simulink model "Clutchless_P2_Parallel_ETE"  (R2017b)
settings: Solver=FixedStepAuto  StartTime=0.0  StopTime=length(Speed)  FixedStep=0.01  MaxStep=0.01  RelTol=1e-3  EnableMultiTasking=on
PostLoadFcn:
  | , if any(exist('dsrtsu_mdlpostloadfcn', 'file') == [2, 3, 6]), try dsrtsu_mdlpostloadfcn('Execute', bdroot); catch fprintf('Error in PostLoadFcn (dsrtsu_mdlpostloadfcn) for model "%s":\n %s\n', bdroot, lasterr); end, end,
undefined symbols (not defined in the file): ABSEnable, Actuators, air, APP1_OOR, APP2_OOR, APP_Mismatch, Brk_Flt, cal, ClutchEngag, Clutchless_HSC_ETE, CS_On_Control, Driver, eng, Engine, EngOverTemp, ENGTRQ_MSMCH_Degraded_CP, ENGTRQ_MSMCH_ErrCritical_CP, ENGTRQ_MSMCH_LimpHome_CP, EngTrqMismatch, env, ess, ESSOverTemp, gb, KeyPos_Flt, KeyPosition, lib_Actuators, lib_Clutchless_HSC_ETE, lib_Driver, lib_EMachine_2017a, lib_Sensors_2017a, LossCAN, Machine, max_vehicle_rad_air_flow, MCUOverTemp, mot, MotDirMismatch, MotOverTemp, MotTrqMismatch, mph2ms, PRNDL_Flt, RegenBrkDisable, RegenFault, Sensors, ShiftLeverPosition, Speed, SW_CS_ON, SW_Engine_ON, t_amb, time, tloop
libraries: simulink x97, Pneumatic_lib x11, nesl_utility x9, EC2_libraries x7, powerlib_meascontrol x2, CalculationGallon x1, lib_Chassis x1, lib_DCDC x1, lib_Differential x1, lib_HVESS x1, fl_lib x1, lib_OBC x1
(part 2 of 9)

== system Clutchless_P2_Parallel_ETE/Camaro Plant Model/E-Machine/Soft MCU ==
  In : Inport
  In1 : Inport  Port=2
  Bus Creator : BusCreator  Inputs=5
  Bus Creator1 : BusCreator  Inputs=2
  Bus Selector : BusSelector  OutputSignals=mot_spd_out,mot_trq_out
  Bus Selector1 : BusSelector  OutputSignals=M192_Command_Message.Inverter_Enable,M192_Command_Message.Torque_Command
  Constant : Constant  Value=0
  Data Type Conversion1 : DataTypeConversion
  Data Type Conversion2 : DataTypeConversion
  Data Type Conversion3 : DataTypeConversion
  ForwardDirection : Constant  Value=0
  Memory : Memory
  Subsystem : Subsystem
  Switch : Switch  Criteria=u2 ~= 0  Threshold=1
  Torque Calculation1 : Subsystem
  Torque Calculation2 : Subsystem  Commented=on
  diff_INV_state : MATLAB Function  TreatAsAtomicUnit=on
  diff_INV_state1 : MATLAB Function  TreatAsAtomicUnit=on
  Out : Outport
  Out1 : Outport  Port=2
  wires:
  In1/1 -> Bus Selector/1, Bus Creator1/2  "Sensors_to_MCU"
  Bus Creator1/1 -> Out/1  "MCU_CAN"
  In/1 -> Bus Selector1/1  "HCU_to_MCU"
  Bus Selector1/2 -> Torque Calculation1/1(MotTrqReq)  "<Torque_Command>"
  Bus Creator/1 -> Bus Creator1/1, Out1/1  "MCU_to _Actuator"
  Constant/1 -> Switch/3
  Bus Selector/1 -> Torque Calculation1/2(MotSpd)  "<mot_spd_out>"
  Data Type Conversion1/1 -> Bus Creator/2  "InverterEnabled"
  Bus Selector/2 -> Torque Calculation1/3(MotTrqFdbck), Data Type Conversion2/1  "<mot_trq_out>"
  Data Type Conversion2/1 -> Bus Creator/3  "MotTrqFdbck"
  Memory/1 -> Data Type Conversion1/1
  Switch/1 -> Data Type Conversion3/1  "MotTrqCmd"
  Data Type Conversion3/1 -> Bus Creator/1  "MotTrqCmd"
  ForwardDirection/1 -> Bus Creator/5  "Direction_Command"
  diff_INV_state/1(y) -> diff_INV_state1/1(u)
  Bus Selector1/1 -> Memory/1, diff_INV_state/1(u)  "<Inverter_Enable>"
  diff_INV_state1/1(y) -> Switch/2
  Torque Calculation1/1(mot_trq_out) -> Switch/1
  Subsystem/1(D3_Power_On_Timer) -> Bus Creator/4

== system Clutchless_P2_Parallel_ETE/Camaro Plant Model/ICE Simple1/Engine Plant Modified ==
  "In " : Inport
  eng_spd_out : Inport  Port=2
  Core Engine : Subsystem
      mask Display: image(imread('EngineShortBlock.jpg'),'center')
  ECU Actuators : Subsystem
  ECU Sensors : Subsystem
  Fuel Supply : Subsystem
      mask Display: image(imread('FuelTank.jpg'),'center')
  Radiator : Subsystem
  Subsystem : Subsystem
  Terminator : Terminator
  Terminator1 : Terminator
  eng_shaft_out : Outport
  Out : Outport  Port=2
  tag scope: EngCrankCmd=global, EngRunAtv=global, EngShutdown=global, Eng_Fan=global, Eng_Temp=global, FuelPumpEnable=global, ThrPstCmd_pct=global, VehSpdAvgDrvn_Eng=global
  wires:
  ECU Actuators/5(Out5) -> [EngShutdown]
  Fuel Supply/1(Available Fuel) -> Core Engine/1(Available Fuel)
  ECU Actuators/4(Out4) -> [FuelPumpEnable]
  ECU Actuators/1(Out1) -> [ThrPstCmd_pct]
  "In "/1 -> ECU Actuators/1(In1)
  ECU Actuators/2(Out2) -> [EngCrankCmd]
  ECU Actuators/3(Out3) -> [EngRunAtv]
  Core Engine/1(eng_shaft_out) -> eng_shaft_out/1
  eng_spd_out/1 -> Core Engine/2(Engine Speed (rad/s))
  [Eng_Fan] -> Radiator/2(Fans)
  [Eng_Temp] -> Radiator/1(EngCltTmp)
  ECU Actuators/6(Out6) -> [Eng_Temp]
  ECU Actuators/7(Out7) -> [Eng_Fan]
  ECU Actuators/8(Out8) -> [VehSpdAvgDrvn_Eng]
  Core Engine/2(Throttle Air Flow (g/s)1) -> Terminator/1  "Throttle Air Flow (g/s)"
  [VehSpdAvgDrvn_Eng] -> Terminator1/1
  [EmsCO] -> ECU Sensors/7(In7)  "CO_g/s"
  ECU Sensors/1(Out1) -> Out/1
  [EmsNOx] -> ECU Sensors/9(In9)  "NOx_g/s"
  [FuelLevelPct] -> ECU Sensors/4(In4)  "FuelLevelPct"
  [AdvFuelFlowEst] -> Subsystem/1(EngFuelFlow_g/s), ECU Sensors/3(In3)  "EngFuelFlow_g/s"
  [EmsHC] -> ECU Sensors/6(In6)  "HC_g/s"
  [EngSpd_RPM] -> ECU Sensors/2(In2)  "EngSpd_RPM"
  [EmsCO2] -> ECU Sensors/8(In8)  "CO2_g/s"
  [EngTemp] -> Subsystem/2(Eng_Temp), ECU Sensors/10(In10)  "Eng_Temp"
  [EngPe] -> ECU Sensors/5(In5)  "PE_0_1"
  [EngBrkTrq] -> ECU Sensors/1(In1)  "EngActStdyStTorq_Nm"

== system Clutchless_P2_Parallel_ETE/Camaro Plant Model/ICE Simple1/Inputs ==
  Analog : Subsystem
  Bus Creator : BusCreator  Inputs=2
  CAN_from_HCU : Subsystem
  Inputs : Outport
  wires:
  CAN_from_HCU/1(Out1) -> Bus Creator/1  "CAN"
  Analog/1(Out1) -> Bus Creator/2  "Analog"
  Bus Creator/1 -> Inputs/1

== system Clutchless_P2_Parallel_ETE/Camaro Plant Model/ICE Simple1/Soft ECM ==
  note: Should check lookup table with GM
  In : Inport
  In1 : Inport  Port=2
  Bus Creator1 : BusCreator  Inputs=3
  Bus Creator2 : BusCreator  Inputs=9
  Bus Selector : BusSelector  OutputSignals=EngSpd_RPM
  Bus Selector1 : BusSelector  OutputSignals=Analog.EngAppReq,CAN.to EBCAN.PPEI_Platform_General_Status.SysPwrMd,CAN.to EBCAN.PPEI_Trans_General_Status_2.TrnsShftLvrPos
  Bus Selector2 : BusSelector  OutputSignals=Eng_Temp
  Bus Selector3 : BusSelector  OutputSignals=EngFuelFlow_g/s
  Data Type Conversion : DataTypeConversion  OutDataTypeStr=int8
  Data Type Conversion1 : DataTypeConversion  OutDataTypeStr=int8
  ECM_RollingAliveCnt : Subsystem
  Fuel Consumption : Subsystem
  Logic : Stateflow chart  TreatAsAtomicUnit=on
  Memory1 : Memory  InitialCondition=Engine.Init_T_amb
  Memory2 : Memory
  temp vs fan : Lookup_n-D  NumberOfTableDimensions=1  BreakpointsForDimension1=[0:1:100]  Table=[0:0.01:1]  InternalRulePriority=Speed  RndMeth=Simplest  InputSameDT=on
  Out : Outport
  Out1 : Outport  Port=2
  tag scope: APP_Eng=global, ShiftLvrPos=global
  wires:
  Logic/3(EngRunAtv) -> Bus Creator2/3  "EngRunAtv"
  Bus Selector/1 -> Logic/4(EngSpd_RPM)  "<EngSpd_RPM>"
  Bus Selector1/1 -> Memory2/1  "<EngAppReq>"
  Logic/2(EngCrankCmd) -> Bus Creator2/2  "Eng12vStrtrMtrCmmdOn"
  Bus Creator1/1 -> Out/1  "ECM_CAN"
  Bus Creator2/1 -> Out1/1, Bus Creator1/1  "ECM_to_Actuators"
  Logic/1(ThrottleCmd) -> Bus Creator2/1  "ThrPosCmd_%"
  In1/1 -> Bus Creator1/3, Bus Selector3/1, Bus Selector2/1, Bus Selector/1  "Sensors_to_ECM"
  Logic/4(FuelPumpEnable) -> Bus Creator2/4  "FuelPumpEnable"
  Bus Selector1/2 -> Data Type Conversion/1  "<SysPwrMd>"
  Bus Selector1/3 -> [ShiftLvrPos], Data Type Conversion1/1  "<TrnsShftLvrPos>"
  Logic/5(EngShutdown) -> Bus Creator2/5  "EngShutdown"
  Bus Selector2/1 -> temp vs fan/1, Memory1/1  "<Eng_Temp>"
  Bus Selector3/1 -> Fuel Consumption/1(Fuel Consumption)  "<EngFuelFlow_g/s>"
  Fuel Consumption/1(fuel consumption) -> Bus Creator1/2  "Eng_fuel_consumption"
  temp vs fan/1 -> Bus Creator2/9  "fan_cmd"
  Memory1/1 -> Bus Creator2/8  "Eng_Temp"
  ECM_RollingAliveCnt/1(Out1) -> Bus Creator2/7
  Data Type Conversion/1 -> Logic/2(SysPwrMd)
  Data Type Conversion1/1 -> Logic/3(ShftLvrPos)
  Memory2/1 -> [APP_Eng], Logic/1(drvAPP)
  In/1 -> Bus Selector1/1  "HCU_to_ECM"
  [VehSpdAvgDrvn] -> Bus Creator2/6, Logic/5(VehSpdAvgDrvn)  "VehSpdAvgDrvn"

== system Clutchless_P2_Parallel_ETE/Camaro Plant Model/Scopes/AxlTrq_to_EngTrq2 ==
  note: //From engine axle torque to engine torque//
  In1 : Inport
  Compare To Constant : simulink/Logic and Bit Operations/Compare To Constant  relop===  const=0  OutDataTypeStr=boolean
  Constant1 : Constant  Value=max(gb.plant.init.ratio.map)
  Constant5 : Constant  Value=fd.plant.init.ratio
  Divide1 : Product  Inputs=*//
  Rate Limiter : RateLimiter  RisingSlewLimit=Engine.trq_uprate  FallingSlewLimit=Engine.trq_derate
  Ratio Filter : Subsystem
  Switch : Switch  Criteria=u2 > Threshold
  Out1 : Outport
  wires:
  In1/1 -> Divide1/1
  Constant5/1 -> Divide1/2
  Divide1/1 -> Rate Limiter/1
  [TransRatio] -> Ratio Filter/1(Ratio)
  Compare To Constant/1 -> Switch/2
  Constant1/1 -> Switch/1
  Switch/1 -> Divide1/3
  Rate Limiter/1 -> Out1/1
  Ratio Filter/1(Filtered_Ratio) -> Switch/3, Compare To Constant/1

== system Clutchless_P2_Parallel_ETE/Camaro Plant Model/Scopes/AxlTrq_to_MtrTrq2 ==
  note: //From motor axle torque to motor torque//
  In1 : Inport
  Compare To Constant : simulink/Logic and Bit Operations/Compare To Constant  relop===  const=0  OutDataTypeStr=boolean
  Constant1 : Constant  Value=max(gb.plant.init.ratio.map)
  Constant5 : Constant  Value=fd.plant.init.ratio
  Divide : Product  Inputs=*//
  Rate Limiter : RateLimiter  RisingSlewLimit=mcu.plant.init.trq_uprate  FallingSlewLimit=mcu.plant.init.trq_derate
  Ratio Filter : Subsystem
  Switch : Switch  Criteria=u2 > Threshold
  Out1 : Outport
  wires:
  In1/1 -> Divide/1
  Constant5/1 -> Divide/2
  Divide/1 -> Rate Limiter/1
  [TransRatio] -> Ratio Filter/1(Ratio)
  Compare To Constant/1 -> Switch/2
  Constant1/1 -> Switch/1
  Rate Limiter/1 -> Out1/1
  Switch/1 -> Divide/3
  Ratio Filter/1(Filtered_Ratio) -> Switch/3, Compare To Constant/1

== system Clutchless_P2_Parallel_ETE/Clutchless_HSC_ETE/HSC/Camaro Fault Detection ==
  Sensors : Inport
  Component Diagnostic : Subsystem
  Input Conversions : Subsystem
  Signal Diagnostic : Subsystem
  SystemDiag : lib_SystemDiag/SystemDiag
  Diagnostic : Outport
  wires:
  Signal Diagnostic/1(SignalDiag) -> Component Diagnostic/1(SignalDiag)
  Component Diagnostic/1(CompDiag) -> SystemDiag/1
  Input Conversions/1(VehSig) -> Signal Diagnostic/1(VehSig)
  Sensors/1 -> Input Conversions/1(RawSig)
  SystemDiag/1 -> Diagnostic/1

== system Clutchless_P2_Parallel_ETE/Clutchless_HSC_ETE/HSC/Driver_Requests ==
  note: Driver management
  Sensors : Inport
  "Diagnostic " : Inport  Port=2
  "Controls " : Inport  Port=3
  APP_BPP to DrvIntndAxlTrq2 : Subsystem
  DriverRequests : Outport
  wires:
  "Controls "/1 -> APP_BPP to DrvIntndAxlTrq2/3(Controls)
  "Diagnostic "/1 -> APP_BPP to DrvIntndAxlTrq2/2(Diag)
  APP_BPP to DrvIntndAxlTrq2/1(IntndAxlTrq) -> DriverRequests/1
  Sensors/1 -> APP_BPP to DrvIntndAxlTrq2/1(Sensors)

== system Clutchless_P2_Parallel_ETE/Clutchless_HSC_ETE/HSC/Powertrain Manager ==
  Sensors : Inport
  Driver Request : Inport  Port=2
  Fault Detection : Inport  Port=3
  Ground : Ground
  HV Manager1 : Subsystem  AncestorBlock=lib_HVManager_PostIMG_2017a/HV Manager
  Output Conversion : Subsystem
  Thermal Manager : Subsystem  AncestorBlock=lib_ThermalManager/Thermal Manager
  Torque Distribution : Subsystem  AncestorBlock=lib_TorqueDistribution_2017a/Torque Distribution
  Out1 : Outport
  Controls : Outport  Port=2
  tag scope: HV_BUS_Status=global
  wires:
  Torque Distribution/1(Controls) -> [Controls], Controls/1, HV Manager1/2(Controls)
  Ground/1 -> Output Conversion/9(In11)  "Trans_test"
  HV Manager1/1(BMS_CAN) -> [BMS_CAN]
  HV Manager1/2(HV_BUS_Status) -> [HV_BUS_Status]
  HV Manager1/4(OBC_Digital) -> [OBC_Digital]
  HV Manager1/3(OBC_CAN) -> [OBC_CAN]
  Driver Request/1 -> Torque Distribution/2(Driver Request)
  [BMS_CAN] -> Output Conversion/1(In1)  "BMS_CAN"
  [OBC_CAN] -> Output Conversion/2(In2)  "OBC_CAN"
  [MCU_CAN] -> Output Conversion/3(In3)  "MCU_CAN"
  [Controls] -> Output Conversion/4(In4)  "Controls"
  Output Conversion/1(Out1) -> Out1/1
  HV Manager1/5(BMS_Digital) -> [BMS_Digital]
  [BMS_Digital] -> Output Conversion/5(In5)  "BMS_Digital"
  Fault Detection/1 -> Torque Distribution/3(Fault Detection)
  Thermal Manager/1(Out1) -> [Fuel_Pump_Control]
  HV Manager1/6(Axiomatic_CAN) -> [Axiomatic_CAN]
  [Axiomatic_CAN] -> Output Conversion/8(In10)  "Axiomatic_CAN"
  [OBC_Digital] -> Output Conversion/7(In9)  "OBC_Digital"
  [Fuel_Pump_Control] -> Output Conversion/6(In8)  "Fuel_Pump_Control"
  Sensors/1 -> Thermal Manager/1(In2), HV Manager1/1(Sensors), Torque Distribution/1(Sensors)

== system Clutchless_P2_Parallel_ETE/Driver/Driver Control/Override CS SW ==
  note: This subsystem is used to override the model value of a signal to a constant value
  note: Override Switch Subsystem
  In1 : Inport
  Multiport Switch : MultiPortSwitch  DataPortOrder=Zero-based contiguous  Inputs=2  zeroidx=on
  Override Value : Constant  Value=0  OutDataTypeStr=double
  Signal Override Switch 0 = Use Model 1 = Use Constant : Constant
  Out1 : Outport
  wires:
  Signal Override Switch 0 = Use Model 1 = Use Constant/1 -> Multiport Switch/1
  In1/1 -> Multiport Switch/2
  Multiport Switch/1 -> Out1/1
  Override Value/1 -> Multiport Switch/3

== system Clutchless_P2_Parallel_ETE/Driver/Driver Control/Override Engine SW ==
  note: Override Switch Subsystem
  note: This subsystem is used to override the model value of a signal to a constant value
  In1 : Inport
  Multiport Switch : MultiPortSwitch  DataPortOrder=Zero-based contiguous  Inputs=2  zeroidx=on
  Override Value : Constant  Value=0  OutDataTypeStr=double
  Signal Override Switch 0 = Use Model 1 = Use Constant : Constant
  Out1 : Outport
  wires:
  Override Value/1 -> Multiport Switch/3
  Multiport Switch/1 -> Out1/1
  In1/1 -> Multiport Switch/2
  Signal Override Switch 0 = Use Model 1 = Use Constant/1 -> Multiport Switch/1

== system Clutchless_P2_Parallel_ETE/Driver/Driver Control/Override Regen SW ==
  note: This subsystem is used to override the model value of a signal to a constant value
  note: Override Switch Subsystem
  In1 : Inport
  Multiport Switch : MultiPortSwitch  DataPortOrder=Zero-based contiguous  Inputs=2  zeroidx=on
  Override Value : Constant  Value=0  OutDataTypeStr=double
  Signal Override Switch 0 = Use Model 1 = Use Constant : Constant
  Out1 : Outport
  wires:
  Signal Override Switch 0 = Use Model 1 = Use Constant/1 -> Multiport Switch/1
  In1/1 -> Multiport Switch/2
  Multiport Switch/1 -> Out1/1
  Override Value/1 -> Multiport Switch/3

== system Clutchless_P2_Parallel_ETE/Fault Trigger /Component Diagnostics setting/Mismch type ==
  In1 : Inport
  Constant : Constant  Value=cal.ENGTRQ_MSMCH.Degraded_CP+1
  Constant1 : Constant  Value=cal.ENGTRQ_MSMCH.LimpHome_CP+1
  Constant2 : Constant  Value=cal.ENGTRQ_MSMCH.ErrCritical_CP+1
  Constant3 : Constant  Value=0
  Multiport Switch : MultiPortSwitch  DataPortOrder=Zero-based contiguous  Inputs=4
  Out1 : Outport
  wires:
  Constant1/1 -> Multiport Switch/4
  Constant2/1 -> Multiport Switch/5
  In1/1 -> Multiport Switch/1
  Multiport Switch/1 -> Out1/1
  Constant3/1 -> Multiport Switch/2
  Constant/1 -> Multiport Switch/3

== system Clutchless_P2_Parallel_ETE/Fault Trigger /Component Diagnostics setting/Mismch type1 ==
  In1 : Inport
  Constant : Constant  Value=cal.MOTTRQ_MSMCH.Degraded_CP+1
  Constant1 : Constant  Value=cal.MOTTRQ_MSMCH.LimpHome_CP+1
  Constant2 : Constant  Value=cal.ENGTRQ_MSMCH.ErrCritical_CP+1
  Constant3 : Constant  Value=0
  Multiport Switch : MultiPortSwitch  DataPortOrder=Zero-based contiguous  Inputs=4
  Out1 : Outport
  wires:
  Constant/1 -> Multiport Switch/3
  Constant3/1 -> Multiport Switch/2
  Multiport Switch/1 -> Out1/1
  In1/1 -> Multiport Switch/1
  Constant2/1 -> Multiport Switch/5
  Constant1/1 -> Multiport Switch/4

== system Clutchless_P2_Parallel_ETE/Fault Trigger /Component Diagnostics setting/Override  ClutchEngag ==
  note: Override Switch Subsystem
  note: This subsystem is used to override the model value of a signal to a constant value
  In1 : Inport
  Constant : Constant  Value=0
  Multiport Switch : MultiPortSwitch  DataPortOrder=Zero-based contiguous  Inputs=2
  Signal Override Switch 0 = Use Model 1 = Use Constant : Constant  Value=ClutchEngagFlt
  Out1 : Outport
  wires:
  Constant/1 -> Multiport Switch/3
  Multiport Switch/1 -> Out1/1
  In1/1 -> Multiport Switch/2
  Signal Override Switch 0 = Use Model 1 = Use Constant/1 -> Multiport Switch/1

== system Clutchless_P2_Parallel_ETE/Fault Trigger /Component Diagnostics setting/Override  ESSOverTemp ==
  note: This subsystem is used to override the model value of a signal to a constant value
  note: Override Switch Subsystem
  In1 : Inport
  Constant : Constant  Value=0
  Multiport Switch : MultiPortSwitch  DataPortOrder=Zero-based contiguous  Inputs=2
  Signal Override Switch 0 = Use Model 1 = Use Constant : Constant  Value=ESSOverTemp_ON
  Out1 : Outport
  wires:
  Signal Override Switch 0 = Use Model 1 = Use Constant/1 -> Multiport Switch/1
  In1/1 -> Multiport Switch/2
  Multiport Switch/1 -> Out1/1
  Constant/1 -> Multiport Switch/3

== system Clutchless_P2_Parallel_ETE/Fault Trigger /Component Diagnostics setting/Override  EngOverTemp ==
  note: Override Switch Subsystem
  note: This subsystem is used to override the model value of a signal to a constant value
  In1 : Inport
  Constant : Constant  Value=0
  Multiport Switch : MultiPortSwitch  DataPortOrder=Zero-based contiguous  Inputs=2
  Signal Override Switch 0 = Use Model 1 = Use Constant : Constant  Value=EngOverTemp_ON
  Out1 : Outport
  wires:
  Constant/1 -> Multiport Switch/3
  Multiport Switch/1 -> Out1/1
  In1/1 -> Multiport Switch/2
  Signal Override Switch 0 = Use Model 1 = Use Constant/1 -> Multiport Switch/1

== system Clutchless_P2_Parallel_ETE/Fault Trigger /Component Diagnostics setting/Override  EngTrqMismatch ==
  note: This subsystem is used to override the model value of a signal to a constant value
  note: Override Switch Subsystem
  In1 : Inport
  Constant : Constant  Value=0
  Multiport Switch : MultiPortSwitch  DataPortOrder=Zero-based contiguous  Inputs=2
  Signal Override Switch 0 = Use Model 1 = Use Constant : Constant  Value=EngTrqMismatch_ON
  Out1 : Outport
  wires:
  Signal Override Switch 0 = Use Model 1 = Use Constant/1 -> Multiport Switch/1
  In1/1 -> Multiport Switch/2
  Multiport Switch/1 -> Out1/1
  Constant/1 -> Multiport Switch/3

== system Clutchless_P2_Parallel_ETE/Fault Trigger /Component Diagnostics setting/Override  LossCAN ==
  note: Override Switch Subsystem
  note: This subsystem is used to override the model value of a signal to a constant value
  In1 : Inport
  Constant : Constant  Value=0
  Multiport Switch : MultiPortSwitch  DataPortOrder=Zero-based contiguous  Inputs=2
  Signal Override Switch 0 = Use Model 1 = Use Constant : Constant  Value=LossCAN_ON
  Out1 : Outport
  wires:
  Constant/1 -> Multiport Switch/3
  Multiport Switch/1 -> Out1/1
  In1/1 -> Multiport Switch/2
  Signal Override Switch 0 = Use Model 1 = Use Constant/1 -> Multiport Switch/1

== system Clutchless_P2_Parallel_ETE/Fault Trigger /Component Diagnostics setting/Override  MCUOverTemp ==
  note: This subsystem is used to override the model value of a signal to a constant value
  note: Override Switch Subsystem
  In1 : Inport
  Constant : Constant  Value=0
  Multiport Switch : MultiPortSwitch  DataPortOrder=Zero-based contiguous  Inputs=2
  Signal Override Switch 0 = Use Model 1 = Use Constant : Constant  Value=MCUOverTemp_ON
  Out1 : Outport
  wires:
  Signal Override Switch 0 = Use Model 1 = Use Constant/1 -> Multiport Switch/1
  In1/1 -> Multiport Switch/2
  Multiport Switch/1 -> Out1/1
  Constant/1 -> Multiport Switch/3

== system Clutchless_P2_Parallel_ETE/Fault Trigger /Component Diagnostics setting/Override  MotDirMismatch ==
  note: Override Switch Subsystem
  note: This subsystem is used to override the model value of a signal to a constant value
  In1 : Inport
  Constant : Constant  Value=0
  Multiport Switch : MultiPortSwitch  DataPortOrder=Zero-based contiguous  Inputs=2
  Signal Override Switch 0 = Use Model 1 = Use Constant : Constant  Value=MotDirMismatch_ON
  Out1 : Outport
  wires:
  Constant/1 -> Multiport Switch/3
  Multiport Switch/1 -> Out1/1
  In1/1 -> Multiport Switch/2
  Signal Override Switch 0 = Use Model 1 = Use Constant/1 -> Multiport Switch/1

== system Clutchless_P2_Parallel_ETE/Fault Trigger /Component Diagnostics setting/Override  MotOverTemp ==
  note: Override Switch Subsystem
  note: This subsystem is used to override the model value of a signal to a constant value
  In1 : Inport
  Constant : Constant  Value=0
  Multiport Switch : MultiPortSwitch  DataPortOrder=Zero-based contiguous  Inputs=2
  Signal Override Switch 0 = Use Model 1 = Use Constant : Constant  Value=MotOverTemp_ON
  Out1 : Outport
  wires:
  Constant/1 -> Multiport Switch/3
  Multiport Switch/1 -> Out1/1
  In1/1 -> Multiport Switch/2
  Signal Override Switch 0 = Use Model 1 = Use Constant/1 -> Multiport Switch/1

== system Clutchless_P2_Parallel_ETE/Fault Trigger /Component Diagnostics setting/Override  MotTrqMismatch ==
  note: This subsystem is used to override the model value of a signal to a constant value
  note: Override Switch Subsystem
  In1 : Inport
  Constant : Constant  Value=0
  Multiport Switch : MultiPortSwitch  DataPortOrder=Zero-based contiguous  Inputs=2
  Signal Override Switch 0 = Use Model 1 = Use Constant : Constant  Value=MotTrqMismatch_ON
  Out1 : Outport
  wires:
  Signal Override Switch 0 = Use Model 1 = Use Constant/1 -> Multiport Switch/1
  In1/1 -> Multiport Switch/2
  Multiport Switch/1 -> Out1/1
  Constant/1 -> Multiport Switch/3

== system Clutchless_P2_Parallel_ETE/Fault Trigger /Driver Interface Diagnostics setting/Override  APP1_OOR ==
  note: Signal Override Switch
      | 0 = Use Model
      | 1 = Use Constant
  note: Override Switch Subsystem
  note: This subsystem is used to override the model value of a signal to a constant value
  In1 : Inport
  APP1_OOR_ON : Constant  Value=APP1_OOR_ON
  Constant : Constant  Value=0
  Multiport Switch : MultiPortSwitch  DataPortOrder=Zero-based contiguous  Inputs=2
  Out1 : Outport
  wires:
  Constant/1 -> Multiport Switch/3
  Multiport Switch/1 -> Out1/1
  In1/1 -> Multiport Switch/2
  APP1_OOR_ON/1 -> Multiport Switch/1

== system Clutchless_P2_Parallel_ETE/Fault Trigger /Driver Interface Diagnostics setting/Override  APP2_OOR ==
  note: Signal Override Switch
      | 0 = Use Model
      | 1 = Use Constant
  note: This subsystem is used to override the model value of a signal to a constant value
  note: Override Switch Subsystem
  In1 : Inport
  APP2_OOR_ON : Constant  Value=APP2_OOR_ON
  Constant : Constant  Value=0
  Multiport Switch : MultiPortSwitch  DataPortOrder=Zero-based contiguous  Inputs=2
  Out1 : Outport
  wires:
  APP2_OOR_ON/1 -> Multiport Switch/1
  In1/1 -> Multiport Switch/2
  Multiport Switch/1 -> Out1/1
  Constant/1 -> Multiport Switch/3

== system Clutchless_P2_Parallel_ETE/Fault Trigger /Driver Interface Diagnostics setting/Override  APP_Mismatch ==
  note: Signal Override Switch
      | 0 = Use Model
      | 1 = Use Constant
  note: Override Switch Subsystem
  note: This subsystem is used to override the model value of a signal to a constant value
  In1 : Inport
  APP_Mismatch_Override : Constant  Value=Mismatch_APP_ON
  Constant : Constant  Value=0
  Multiport Switch : MultiPortSwitch  DataPortOrder=Zero-based contiguous  Inputs=2
  Out1 : Outport
  wires:
  Constant/1 -> Multiport Switch/3
  Multiport Switch/1 -> Out1/1
  In1/1 -> Multiport Switch/2
  APP_Mismatch_Override/1 -> Multiport Switch/1

== system Clutchless_P2_Parallel_ETE/Fault Trigger /Driver Interface Diagnostics setting/Override  BPP_Flt ==
  note: Signal Override Switch
      | 0 = Use Model
      | 1 = Use Constant
  note: This subsystem is used to override the model value of a signal to a constant value
  note: Override Switch Subsystem
  In1 : Inport
  Brk_Flt_ON : Constant  Value=Brk_Flt_ON
  Constant : Constant  Value=0
  Multiport Switch : MultiPortSwitch  DataPortOrder=Zero-based contiguous  Inputs=2
  Out1 : Outport
  wires:
  Brk_Flt_ON/1 -> Multiport Switch/1
  In1/1 -> Multiport Switch/2
  Multiport Switch/1 -> Out1/1
  Constant/1 -> Multiport Switch/3

== system Clutchless_P2_Parallel_ETE/Fault Trigger /Driver Interface Diagnostics setting/Override  KeyPos_Flt ==
  note: Signal Override Switch
      | 0 = Use Model
      | 1 = Use Constant
  note: Override Switch Subsystem
  note: This subsystem is used to override the model value of a signal to a constant value
  In1 : Inport
  Constant : Constant  Value=0
  KeyPos_Flt_ON : Constant  Value=KeyPos_Flt_ON
  Multiport Switch : MultiPortSwitch  DataPortOrder=Zero-based contiguous  Inputs=2
  Out1 : Outport
  wires:
  Constant/1 -> Multiport Switch/3
  Multiport Switch/1 -> Out1/1
  In1/1 -> Multiport Switch/2
  KeyPos_Flt_ON/1 -> Multiport Switch/1

== system Clutchless_P2_Parallel_ETE/Fault Trigger /Driver Interface Diagnostics setting/Override  PRNDL_Flt ==
  note: Signal Override Switch
      | 0 = Use Model
      | 1 = Use Constant
  note: This subsystem is used to override the model value of a signal to a constant value
  note: Override Switch Subsystem
  In1 : Inport
  Constant : Constant  Value=0
  Multiport Switch : MultiPortSwitch  DataPortOrder=Zero-based contiguous  Inputs=2
  PRNDL_Flt_ON : Constant  Value=PRNDL_Flt_ON
  Out1 : Outport
  wires:
  PRNDL_Flt_ON/1 -> Multiport Switch/1
  In1/1 -> Multiport Switch/2
  Multiport Switch/1 -> Out1/1
  Constant/1 -> Multiport Switch/3

== system Clutchless_P2_Parallel_ETE/Sensors/CAN/EBCAN ==
  In1 : Inport
  BMS_Antrieb : Subsystem
  Bus Creator : BusCreator  Inputs=3
  Bus Selector : BusSelector  OutputSignals=ECM_CAN,BMS_CAN.BMS_Hybrid
  CCM : Subsystem
  ECM : Subsystem
  Out1 : Outport
  wires:
  Bus Selector/2 -> CCM/1(In1), BMS_Antrieb/1(In1)  "<BMS_Hybrid>"
  Bus Selector/1 -> ECM/1(In1)  "<ECM_CAN>"
  In1/1 -> Bus Selector/1
  CCM/1(Out1) -> Bus Creator/3  "from_CCM"
  Bus Creator/1 -> Out1/1
  BMS_Antrieb/1(Out1) -> Bus Creator/2  "from_BMSAntrieb"
  ECM/1(Out1) -> Bus Creator/1  "from_ECM"

== system Clutchless_P2_Parallel_ETE/Sensors/CAN/HV_CAN ==
  In1 : Inport
  BMS_Hybrid : Subsystem
  Bus Creator : BusCreator  Inputs=3
  Bus Selector : BusSelector  OutputSignals=MCU_CAN,BMS_CAN.BMS_Plugin,OBC_CAN
  MCU : Subsystem
  OBC : Subsystem
  Out1 : Outport
  wires:
  Bus Selector/3 -> OBC/1(In1)  "<OBC_CAN>"
  Bus Selector/2 -> BMS_Hybrid/1(In1)  "<BMS_Plugin>"
  Bus Selector/1 -> MCU/1(In1)  "<MCU_CAN>"
  In1/1 -> Bus Selector/1
  Bus Creator/1 -> Out1/1
  OBC/1(Out1) -> Bus Creator/3  "from_OBC"
  BMS_Hybrid/1(Out1) -> Bus Creator/2  "from_BMSHybrid"
  MCU/1(Out1) -> Bus Creator/1  "from_MCU"

== system Clutchless_P2_Parallel_ETE/Sensors/CAN/VEH_CAN ==
  In1 : Inport
  BCM : Subsystem
  Bus Creator : BusCreator  Inputs=4
  Bus Selector : BusSelector  OutputSignals=TCM_CAN,BCM_CAN
  EBCM : Subsystem  Commented=on
  Ground : Ground  Commented=on
  Ground1 : Ground  Commented=on
  ICCM : Subsystem  Commented=on
  TCM : Subsystem
  Out1 : Outport
  wires:
  Ground/1 -> EBCM/1(In1)  "<EBCM>"
  Ground1/1 -> ICCM/1(In1)  "<ONSTAR>"
  Bus Selector/2 -> BCM/1(In1)  "<BCM_CAN>"
  Bus Selector/1 -> TCM/1(In1)  "<TCM_CAN>"
  Bus Creator/1 -> Out1/1
  EBCM/1(Out1) -> Bus Creator/4  "from_EBCM"
  ICCM/1(Out1) -> Bus Creator/3  "from_ICCM"
  BCM/1(Out1) -> Bus Creator/2  "from_BCM"
  TCM/1(Out1) -> Bus Creator/1  "from_TCM"
  In1/1 -> Bus Selector/1

== system Clutchless_P2_Parallel_ETE/Actuators/CAN/EBCAN/ISO_Hybrid_01_Req ==
  In1 : Inport
  Bus Creator : BusCreator  Inputs=1
  Bus Selector : BusSelector  OutputSignals=ISO_Hybrid_01_Req_Data_byte_3
  Data Type Conversion : DataTypeConversion
  Out1 : Outport
  wires:
  In1/1 -> Bus Selector/1
  Data Type Conversion/1 -> Bus Creator/1  "ISO_Hybrid_01_Req_Data_4"
  Bus Creator/1 -> Out1/1  "ISO_Hybrid_01_Req"
  Bus Selector/1 -> Data Type Conversion/1  "<ISO_Hybrid_01_Req_Data_byte_3>"

== system Clutchless_P2_Parallel_ETE/Actuators/CAN/EBCAN/PPEI_Platform_General_Status ==
  In1 : Inport
  Bus Creator : BusCreator  Inputs=1
  Data Type Conversion : DataTypeConversion
  Out1 : Outport
  wires:
  Bus Creator/1 -> Out1/1  "PPEI_Platform_General_Status"
  Data Type Conversion/1 -> Bus Creator/1  "SysPwrMd"
  In1/1 -> Data Type Conversion/1

== system Clutchless_P2_Parallel_ETE/Actuators/CAN/EBCAN/PPEI_Trans_General_Status_2 ==
  In1 : Inport
  Bus Creator : BusCreator  Inputs=1
  Data Type Conversion : DataTypeConversion
  Out1 : Outport
  wires:
  In1/1 -> Data Type Conversion/1
  Data Type Conversion/1 -> Bus Creator/1  "TrnsShftLvrPos"
  Bus Creator/1 -> Out1/1  "PPEI_Trans_General_Status_2"

== system Clutchless_P2_Parallel_ETE/Actuators/CAN/VEH_CAN/BCM ==
  In1 : Inport
  Bus Creator : BusCreator  Inputs=1
  Bus Selector : BusSelector  OutputSignals=Controls.powerMode
  Out1 : Outport
  wires:
  In1/1 -> Bus Selector/1
  Bus Selector/1 -> Bus Creator/1  "<powerMode>"
  Bus Creator/1 -> Out1/1

== system Clutchless_P2_Parallel_ETE/Actuators/CAN/VEH_CAN/EBCM ==
  In1 : Inport
  Out1 : Outport
  wires:
  In1/1 -> Out1/1

== system Clutchless_P2_Parallel_ETE/Actuators/CAN/VEH_CAN/ICCM ==
  In1 : Inport
  Out1 : Outport
  wires:
  In1/1 -> Out1/1

== system Clutchless_P2_Parallel_ETE/Camaro Plant Model/E-Machine/IMG Plant/ Actuators ==
  In1 : Inport
  Bus Selector : BusSelector  OutputSignals=MotTrqCmd,Direction_Command,InverterEnabled
  MotTrqCmd : Outport
  DirectionCommand : Outport  Port=2
  InverterEnabled : Outport  Port=3
  wires:
  In1/1 -> Bus Selector/1
  Bus Selector/1 -> MotTrqCmd/1  "<MotTrqCmd>"
  Bus Selector/2 -> DirectionCommand/1  "<Direction_Command>"
  Bus Selector/3 -> InverterEnabled/1  "<InverterEnabled>"

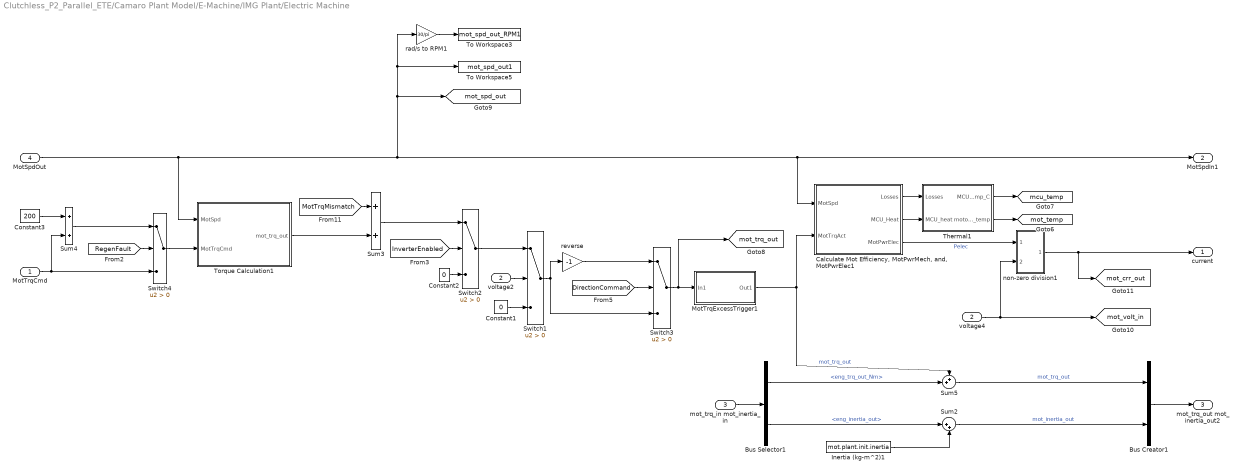
== system Clutchless_P2_Parallel_ETE/Camaro Plant Model/E-Machine/IMG Plant/Electric Machine ==
  MotTrqCmd : Inport
  voltage2 : Inport  Port=2
  mot_trq_in mot_inertia_in : Inport  Port=3
  MotSpdOut : Inport  Port=4
  Bus Creator1 : BusCreator  Inputs=2
  Bus Selector1 : BusSelector  OutputSignals=eng_trq_out_Nm,eng_inertia_out
  "Calculate Mot Efficiency, MotPwrMech, and, MotPwrElec1" : Subsystem
  Constant1 : Constant  Value=0
  Constant2 : Constant  Value=0
  Constant3 : Constant  Value=200
  Inertia (kg-m^2)1 : Constant  Value=mot.plant.init.inertia
  MotTrqExcessTrigger1 : Subsystem
  Sum2 : Sum  Inputs=|++
  Sum3 : Sum
  Sum4 : Sum
  Sum5 : Sum  Inputs=++|
  Switch{1..4} (4 alike) : Switch  Criteria=u2 > Threshold
  Thermal1 : Subsystem
  To Workspace3 : ToWorkspace  VariableName=mot_spd_out_RPM1  SampleTime=-1
      settings: Decimation=WORKSPACE_DECIMATION
  To Workspace5 : ToWorkspace  VariableName=mot_spd_out1  SampleTime=-1
      settings: Decimation=WORKSPACE_DECIMATION
  Torque Calculation1 : Subsystem
  non-zero division1 : Subsystem
      mask Display: disp('divider \n I1/I2')
  rad/s to RPM1 : Gain  Gain=30/pi
  reverse : Gain  Gain=-1
  voltage4 : InportShadow  Port=2
  current : Outport
  MotSpdIn1 : Outport  Port=2
  mot_trq_out mot_inertia_out2 : Outport  Port=3
  tag scope: mcu_temp=global, mot_crr_out=global, mot_spd_out=global, mot_temp=global, mot_trq_out=global, mot_volt_in=global
  wires:
  Thermal1/1(MCU_temp_C) -> [mcu_temp]
  Thermal1/2(motor_temp) -> [mot_temp]
  Constant3/1 -> Sum4/1
  Torque Calculation1/1(mot_trq_out) -> Sum3/2
  Switch2/1 -> Switch1/1
  [RegenFault] -> Switch4/2
  "Calculate Mot Efficiency, MotPwrMech, and, MotPwrElec1"/1(Losses) -> Thermal1/1(Losses)
  Sum4/1 -> Switch4/1
  Switch3/1 -> MotTrqExcessTrigger1/1(In1), [mot_trq_out]
  "Calculate Mot Efficiency, MotPwrMech, and, MotPwrElec1"/2(MCU_Heat) -> Thermal1/2(MCU_heat)
  Switch4/1 -> Torque Calculation1/2(MotTrqCmd)
  "Calculate Mot Efficiency, MotPwrMech, and, MotPwrElec1"/3(MotPwrElec) -> non-zero division1/1(In1)  "Pelec"
  reverse/1 -> Switch3/1
  non-zero division1/1(Out1) -> [mot_crr_out], current/1
  MotTrqExcessTrigger1/1(Out1) -> Sum5/1, "Calculate Mot Efficiency, MotPwrMech, and, MotPwrElec1"/2(MotTrqAct)  "mot_trq_out"
  Sum3/1 -> Switch2/1
  MotTrqCmd/1 -> Sum4/2, Switch4/3
  Constant2/1 -> Switch2/3
  Switch1/1 -> reverse/1, Switch3/3
  Constant1/1 -> Switch1/3
  voltage2/1 -> Switch1/2
  voltage4/1 -> non-zero division1/2(In2), [mot_volt_in]
  [MotTrqMismatch] -> Sum3/1
  [InverterEnabled] -> Switch2/2
  [DirectionCommand] -> Switch3/2
  Sum5/1 -> Bus Creator1/1  "mot_trq_out"
  Inertia (kg-m^2)1/1 -> Sum2/2
  Sum2/1 -> Bus Creator1/2  "mot_inertia_out"
  Bus Creator1/1 -> mot_trq_out mot_inertia_out2/1
  mot_trq_in mot_inertia_in/1 -> Bus Selector1/1
  Bus Selector1/2 -> Sum2/1  "<eng_inertia_out>"
  Bus Selector1/1 -> Sum5/2  "<eng_trq_out_Nm>"
  rad/s to RPM1/1 -> To Workspace3/1
  MotSpdOut/1 -> "Calculate Mot Efficiency, MotPwrMech, and, MotPwrElec1"/1(MotSpd), MotSpdIn1/1, To Workspace5/1, rad/s to RPM1/1, [mot_spd_out], Torque Calculation1/1(MotSpd)

== system Clutchless_P2_Parallel_ETE/Camaro Plant Model/E-Machine/IMG Plant/Sensors ==
  In2 : Inport
  In3 : Inport  Port=2
  In4 : Inport  Port=3
  In5 : Inport  Port=4
  In6 : Inport  Port=5
  In1 : Inport  Port=6
  In7 : Inport  Port=7
  Bus Creator : BusCreator  Inputs=7
  Out1 : Outport
  wires:
  Bus Creator/1 -> Out1/1
  In2/1 -> Bus Creator/1  "mot_spd_out"
  In4/1 -> Bus Creator/3  "mot_crr_out"
  In5/1 -> Bus Creator/4  "mot_volt_in"
  In3/1 -> Bus Creator/2  "mot_trq_out"
  In6/1 -> Bus Creator/5  "mot_temp"
  In1/1 -> Bus Creator/6  "mcu_temp"
  In7/1 -> Bus Creator/7  "clt_plant_spd_in"

== system Clutchless_P2_Parallel_ETE/Camaro Plant Model/E-Machine/IMG Plant2/ Actuators ==
  In1 : Inport
  Bus Selector : BusSelector  OutputSignals=MotTrqCmd,Direction_Command,InverterEnabled
  Out2 : Outport
  Out3 : Outport  Port=2
  Out4 : Outport  Port=3
  wires:
  Bus Selector/3 -> Out4/1  "<InverterEnabled>"
  Bus Selector/2 -> Out3/1  "<Direction_Command>"
  In1/1 -> Bus Selector/1
  Bus Selector/1 -> Out2/1  "<MotTrqCmd>"

== system Clutchless_P2_Parallel_ETE/Camaro Plant Model/E-Machine/IMG Plant2/Calculate Mot Efficiency, MotPwrMech, and, MotPwrElec ==
  note: Pelec_req = Pmech_req*Eff^k,
      | k = -1 if Trq >= 0,
      | k = 1 if Trq < 0
  MotSpd : Inport
  MotTrqAct : Inport  Port=2
  -1 : Gain  Gain=8
  "-1 when + 1 when - " : Gain  Gain=-1
  -2 : Gain  Gain=tloop
  2-D Lookup Table : Lookup_n-D  BreakpointsForDimension1=mot.plant.init.eff_trq.idx2_trq  BreakpointsForDimension2=mot.plant.init.eff_trq.idx1_spd  Table=mot.plant.init.eff_trq.map  InternalRulePriority=Speed  RndMeth=Simplest  InputSameDT=on
  Abs{,1..3} (4 alike) : Abs
  Add : Sum  Inputs=-+
  Add1 : Sum  Inputs=+-
  Add2 : Sum  Commented=on
  Constant : Constant  Value=1-0.8
  Constant1 : Constant  Commented=on  Value=mot.plant.init.mcu_mass
  Constant2 : Constant  Commented=on  Value=mot.plant.init.specific_heat
  Divide : Product  Commented=on  Inputs=*/
  Gain2 : Gain  Gain=1/100
  Lower Limit : Subsystem  Commented=on  mask{Lolimit=t_amb+20}
      mask prompts: Lolimit "Lower Limit"
  MCUOverTemp Fault : Subsystem  Commented=on
  MCU_WEGPmp : Constant  Value=0
  Math Function1 : Math  Operator=pow  SaturateOnIntegerOverflow=on
  Memory : Memory
  Memory1 : Memory  Commented=on
  Product : Product
  Product1 : Product
  Product2 : Product
  Product3 : Product  Commented=on
  Sign : Signum
  rad/s to rpm : Gain  Gain=30/pi
  Losses : Outport
  MotPwrElec : Outport  Port=2
  MCU_Heat : Outport  Port=3
  wires:
  Lower Limit/1(Out1) -> Memory1/1, MCUOverTemp Fault/1(In1)
  Add2/1 -> Lower Limit/1(In1)
  Memory1/1 -> Add2/2
  Divide/1 -> Add2/1
  Product3/1 -> Divide/2
  Constant2/1 -> Product3/2
  Constant1/1 -> Product3/1
  -2/1 -> MCU_Heat/1
  -1/1 -> Add1/2
  Add1/1 -> -2/1
  MCU_WEGPmp/1 -> -1/1
  Abs3/1 -> Add1/1
  Product2/1 -> Abs3/1
  Constant/1 -> Product2/2
  Memory/1 -> Sign/1
  Math Function1/1 -> Product1/2
  Add/1 -> Abs2/1
  Abs2/1 -> Losses/1
  "-1 when + 1 when - "/1 -> Math Function1/2
  MotSpd/1 -> rad/s to rpm/1, Product/2
  MotTrqAct/1 -> Abs/1, Product/1, Memory/1
  Product/1 -> Product1/1, Add/1  "MotPwrMech"
  Product1/1 -> MotPwrElec/1, Add/2, Product2/1  "MotPwrElec"
  2-D Lookup Table/1 -> Gain2/1
  Gain2/1 -> Math Function1/1
  Abs/1 -> 2-D Lookup Table/1
  Sign/1 -> "-1 when + 1 when - "/1
  Abs1/1 -> 2-D Lookup Table/2
  rad/s to rpm/1 -> Abs1/1

== system Clutchless_P2_Parallel_ETE/Camaro Plant Model/E-Machine/IMG Plant2/MotTrqExcessTrigger ==
  In1 : Inport
  Bias : Bias  Bias=55
  Bias1 : Bias  Bias=25
  Constant : Constant  Value=0
  Multiport Switch : MultiPortSwitch  DataPortOrder=Zero-based contiguous
  Out1 : Outport
  tag scope: MotTrqExcessTrig=global
  wires:
  Constant/1 -> Multiport Switch/1, [MotTrqExcessTrig]
  Bias1/1 -> Multiport Switch/3
  In1/1 -> Bias1/1, Bias/1, Multiport Switch/2
  Bias/1 -> Multiport Switch/4
  Multiport Switch/1 -> Out1/1

== system Clutchless_P2_Parallel_ETE/Camaro Plant Model/E-Machine/IMG Plant2/Motor_Plant ==
  Trq_cmd : Inport
  Batt_volt : Inport  Port=2
  Speed_rad/sec : Inport  Port=3
  Add : Sum
  Bus Creator : BusCreator  Inputs=5
  Efficiency Calcs : Subsystem
  Memory : Memory
  Random Number : RandomNumber  Mean=0.1  Variance=0.1  SampleTime=0.01
  rad/sec to rpm : Gain  Gain=60/(2*3.14)
  Mot_out : Outport
  wires:
  Efficiency Calcs/3(Elec_power_W) -> Bus Creator/5
  Efficiency Calcs/2(Mech_power_W) -> Bus Creator/4
  Efficiency Calcs/1(Mot_current) -> Bus Creator/3
  Batt_volt/1 -> Efficiency Calcs/3(Batt_volt)
  Trq_cmd/1 -> Add/1
  Bus Creator/1 -> Mot_out/1
  Memory/1 -> Efficiency Calcs/2(Torq_cmd_Nm), Bus Creator/1  "Mot_Trq_Nm"
  Random Number/1 -> Add/2
  rad/sec to rpm/1 -> Efficiency Calcs/1(Speed_rpm), Bus Creator/2  "Mot_spd_rpm"
  Speed_rad/sec/1 -> rad/sec to rpm/1
  Add/1 -> Memory/1

== system Clutchless_P2_Parallel_ETE/Camaro Plant Model/E-Machine/IMG Plant2/Sensors ==
  In2 : Inport
  In3 : Inport  Port=2
  In4 : Inport  Port=3
  In5 : Inport  Port=4
  In6 : Inport  Port=5
  In1 : Inport  Port=6
  In7 : Inport  Port=7
  Bus Creator : BusCreator  Inputs=7
  Out1 : Outport
  wires:
  In7/1 -> Bus Creator/7  "clt_plant_spd_in"
  In1/1 -> Bus Creator/6  "mcu_temp"
  Bus Creator/1 -> Out1/1
  In2/1 -> Bus Creator/1  "mot_spd_out"
  In4/1 -> Bus Creator/3  "mot_crr_out"
  In5/1 -> Bus Creator/4  "mot_volt_in"
  In3/1 -> Bus Creator/2  "mot_trq_out"
  In6/1 -> Bus Creator/5  "mot_temp"

== system Clutchless_P2_Parallel_ETE/Camaro Plant Model/E-Machine/IMG Plant2/Thermal ==
  Losses : Inport
  Motor Thermal : Subsystem
  mot_temp_C : Outport
  wires:
  Motor Thermal/1(Out1) -> mot_temp_C/1
  Losses/1 -> Motor Thermal/1(In1)  "[W]"

== system Clutchless_P2_Parallel_ETE/Camaro Plant Model/E-Machine/IMG Plant2/Thermal1 ==
  Losses : Inport
  MCU_heat : Inport  Port=2
  MotInv_loop : Subsystem
  Motor Thermal : Subsystem  Commented=on
  MCU_temp_C : Outport
  motor_temp : Outport  Port=2
  wires:
  MotInv_loop/2(Out2) -> motor_temp/1
  MotInv_loop/1(Out1) -> MCU_temp_C/1
  Losses/1 -> MotInv_loop/1(In1)  "[W]"
  MCU_heat/1 -> MotInv_loop/2(In2)

== system Clutchless_P2_Parallel_ETE/Camaro Plant Model/E-Machine/IMG Plant2/Torque Calculation ==
  MotSpd : Inport
  MotTrqCmd : Inport  Port=2
  Abs : Abs
  Abs1 : Abs
  MinMax : MinMax  Inputs=2
  Product : Product
  Sign : Signum
  electric machine filter : Subsystem
  "max torque " : Subsystem
  mot_trq_out : Outport
  wires:
  Product/1 -> electric machine filter/1(trq)
  MotTrqCmd/1 -> Abs/1, Sign/1, "max torque "/1(cmd)
  electric machine filter/1(filtered) -> mot_trq_out/1
  Abs1/1 -> MinMax/2
  Abs/1 -> MinMax/1
  MinMax/1 -> Product/2
  Sign/1 -> Product/1
  MotSpd/1 -> "max torque "/2(speed)
  "max torque "/1(max torque) -> Abs1/1

== system Clutchless_P2_Parallel_ETE/Camaro Plant Model/E-Machine/IMG Plant2/non-zero division ==
  note: and finally, the expression is: (u[1] \ u[2]) * 1 = u[1] \ u[2]
  note: (u[2]!=0) is true then returns 1
  note: if u[2] != 0, then output == u[1]\u[2]:
  note: (u[2]==0) is false then returns 0, thus (u[2]+(u[2]==0)) is equal to u[2]+0=u[2]
  note: and finally, the expression is: (u[1] \ 1) * 0 = 0
  note: (u[2]!=0) is false then returns 0
  note: if u[2] == 0, then output == 0:
  note: (u[2]==0) is true then returns 1, thus (u[2]+(u[2]==0)) is equal to 0+1=1
  note: original idea from Phil Sharer - ANL
      | original formula: u[1]\(u[2]+eps)*(u[2]!=0)
      | changes done by Gerald ZINI (dgey) - ANL (05\02\2001)
  In1 : Inport
  In2 : Inport  Port=2
  Fcn : Fcn  Expr=u[1]/(u[2]+(u[2]==0))*(u[2]!=0)
  Mux : Mux  Inputs=2
  Out1 : Outport
  wires:
  In2/1 -> Mux/2
  Fcn/1 -> Out1/1
  In1/1 -> Mux/1
  Mux/1 -> Fcn/1

== system Clutchless_P2_Parallel_ETE/Camaro Plant Model/E-Machine/Soft MCU/Subsystem ==
  MCU_RollingAliveCnt : Subsystem
  D3_Power_On_Timer : Outport
  wires:
  MCU_RollingAliveCnt/1(Out1) -> D3_Power_On_Timer/1  "D3_Power_On_Timer"

== system Clutchless_P2_Parallel_ETE/Camaro Plant Model/E-Machine/Soft MCU/Torque Calculation1 ==
  MotTrqReq : Inport
  MotSpd : Inport  Port=2
  MotTrqFdbck : Inport  Port=3
  Abs : Abs
  Abs1 : Abs
  MinMax : MinMax  Inputs=2
  Product : Product
  Sign : Signum
  "max torque " : Subsystem
  mot_trq_out : Outport
  wires:
  Product/1 -> mot_trq_out/1
  "max torque "/1(max torque) -> Abs1/1
  MotSpd/1 -> "max torque "/2(speed)
  MotTrqReq/1 -> "max torque "/1(Req), Sign/1, Abs/1
  Sign/1 -> Product/1
  MinMax/1 -> Product/2
  Abs/1 -> MinMax/1
  Abs1/1 -> MinMax/2
  MotTrqFdbck/1 -> "max torque "/3(torque)

== system Clutchless_P2_Parallel_ETE/Camaro Plant Model/E-Machine/Soft MCU/Torque Calculation2 ==
  MotTrqReq : Inport
  MotSpd : Inport  Port=2
  MotTrqFdbck : Inport  Port=3
  mot_temp : Inport  Port=4
  mcu_temp : Inport  Port=5
  mot_volt_in : Inport  Port=6
  1-D Lookup Table : Lookup_n-D  NumberOfTableDimensions=1  BreakpointsForDimension1=[0,12600,12700,12800,12900,13000]  Table=[1,1,0.75,0.5,0.25,0]  InternalRulePriority=Speed  RndMeth=Simplest  InputSameDT=on
  1-D Lookup Table1 : Lookup_n-D  NumberOfTableDimensions=1  BreakpointsForDimension1=[0,410,415,420,425,430]  Table=[1,1,0.75,0.5,0.25,0]  InternalRulePriority=Speed  RndMeth=Simplest  InputSameDT=on
  1-D Lookup Table2 : Lookup_n-D  Commented=on  NumberOfTableDimensions=1  BreakpointsForDimension1=[0,90,100]  Table=[1,1,0]  InternalRulePriority=Speed  RndMeth=Simplest  InputSameDT=on
  1-D Lookup Table3 : Lookup_n-D  NumberOfTableDimensions=1  BreakpointsForDimension1=[0,150,170]  Table=[1,1,0]  InternalRulePriority=Speed  RndMeth=Simplest  InputSameDT=on
  Abs : Abs
  Abs1 : Abs
  Constant : Constant
  MinMax : MinMax  Inputs=2
  Product : Product
  Product1 : Product  Inputs=5
  Sign : Signum
  Terminator1 : Terminator
  "max torque " : Subsystem
  rad/s to RPM1 : Gain  Gain=30/pi
  mot_trq_out : Outport
  wires:
  Product/1 -> Product1/5
  "max torque "/1(max torque) -> Abs1/1
  MotSpd/1 -> rad/s to RPM1/1, "max torque "/2(speed)
  MotTrqReq/1 -> "max torque "/1(Req), Sign/1, Abs/1
  Sign/1 -> Product/1
  MinMax/1 -> Product/2
  Abs/1 -> MinMax/1
  Abs1/1 -> MinMax/2
  MotTrqFdbck/1 -> "max torque "/3(torque)
  rad/s to RPM1/1 -> 1-D Lookup Table/1
  Product1/1 -> mot_trq_out/1
  1-D Lookup Table/1 -> Product1/4
  mot_volt_in/1 -> 1-D Lookup Table1/1
  1-D Lookup Table1/1 -> Product1/3
  mot_temp/1 -> 1-D Lookup Table3/1
  mcu_temp/1 -> Terminator1/1
  Constant/1 -> Product1/2
  1-D Lookup Table3/1 -> Product1/1

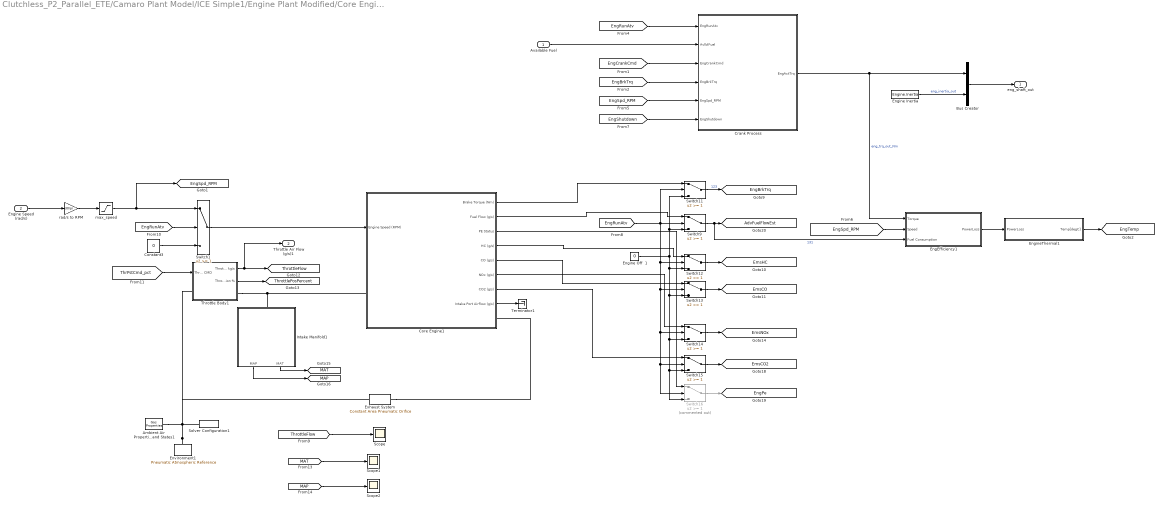
== system Clutchless_P2_Parallel_ETE/Camaro Plant Model/ICE Simple1/Engine Plant Modified/Core Engine ==
  Available Fuel : Inport
  Engine Speed (rad/s) : Inport  Port=2
  Ambient Air Properties and States1 : Pneumatic_lib/Pneumatic Utilities/Gas Properties  c_p=1.005e+3 J/kg/K  c_v=717.95 J/kg/K  viscosity=1.821e-5 s*Pa  Pa=100 kPa  Ta=293.15 K  range_error=1
  Bus Creator : BusCreator  Inputs=2
  Constant3 : Constant  Value=0
  Core Engine1 : Subsystem
      mask Display: image(imread('EngineShortBlock.jpg'),'center')
  Crank Process : Stateflow chart  TreatAsAtomicUnit=on
  EngEfficiency1 : Subsystem
  Engine Inertia : Constant  Value=Engine.Inertia
  Engine Off  1 : Constant  Value=0
  EngineThermal1 : Subsystem
  Environment1 : Pneumatic_lib/Pneumatic Elements/Pneumatic Atmospheric Reference
  Exhaust System : Pneumatic_lib/Pneumatic Elements/Constant Area Pneumatic Orifice  Cd=0.8  Area=0.25*pi*(4*0.0254)^2 m^2  G_specify=off  G_priority=High  G=0 kg/s  G_nominal_specify=off  G_nominal_unit=kg/s  G_nominal_value=1  Q1_specify=off  Q1_priority=High  Q1=0 J/s  Q1_nominal_specify=off  Q1_nominal_unit=J/s  Q1_nominal_value=1  Q2_specify=off  Q2_priority=High  Q2=0 J/s  Q2_nominal_specify=off  Q2_nominal_unit=J/s  Q2_nominal_value=1  p1_specify=off  p1_priority=High  p1=1e+5 Pa  p1_nominal_specify=off  p1_nominal_unit=Pa  p1_nominal_value=1  p2_specify=off  p2_priority=High  p2=1e+5 Pa  p2_nominal_specify=off  p2_nominal_unit=Pa  p2_nominal_value=1  T1_specify=off  T1_priority=High  T1=300 K  T1_nominal_specify=off  T1_nominal_unit=K  T1_nominal_value=1  T2_specify=off  T2_priority=High  T2=300 K  T2_nominal_specify=off  T2_nominal_unit=K  T2_nominal_value=1
  Intake Manifold1 : Subsystem
      mask Display: image(imread('IntakeManifold.jpg'),'center')
  Scope : Scope
  Scope1 : Scope
  Scope2 : Scope
  Solver Configuration1 : nesl_utility/Solver Configuration  PhysicalDomain=network_engine_domain  SubClassName=solver  LeftPortType=input  RightPortType=generic  Accelerate=off  Tones=[]  Harmonics=[]  SimulateNoise=off  Profile=off  UseLocalSampling=off  EnableSwitchedLinearOptims=on  FrequencyDomain=off  UseCCode=off  RelTol=0.001  AbsTol=1e-06  MinStep=1e-09  ToWorkspace=off  RevertToSquareIcSolve=off  NumHomotopyIterations=100  PhasorMode=off  PhasorModeNumHarmonics=1  DoDC=off  ResidualTolerance=1e-9  UseLocalSolver=on  LocalSolverChoice=NE_BACKWARD_EULER_ADVANCER  LocalSolverSampleTime=.01  DoFixedCost=off  MaxNonlinIter=3  MaxModeIter=2  LinearAlgebra=Sparse  DelaysMemoryBudget=1024  AutomaticFiltering=on  FilteringTimeConstant=0.001
  Switch{1,9,11..15} (7 alike) : Switch  Threshold=1
  Switch16 : Switch  Commented=on  Threshold=1
  Terminator1 : Terminator
  Throttle Body1 : Subsystem
      mask Display: image(imread('ElectronicThrottle.jpg'),'center')
  max_speed : Saturate  UpperLimit=max(Engine.Engine.TQ.SPEED)  LowerLimit=0
  rad/s to RPM : Gain  Gain=30/pi
  eng_shaft_out : Outport
  Throttle Air Flow (g/s)1 : Outport  Port=2
  tag scope: AdvFuelFlowEst=global, EmsCO2=global, EmsCO=global, EmsHC=global, EmsNOx=global, EngBrkTrq=global, EngPe=global, EngSpd_RPM=global, EngTemp=global, MAP=global, MAT=global, ThrottleFlow=global, ThrottlePosPercent=global
  wires:
  Throttle Body1/2(Throttle Position %) -> [ThrottlePosPercent]
  Core Engine1/8(Intake Port Airflow (g/s)) -> Terminator1/1
  Intake Manifold1/1(MAP) -> [MAP]
  Intake Manifold1/2(MAT) -> [MAT]
  Throttle Body1/1(Throttle Flow kg/s) -> Throttle Air Flow (g/s)1/1, [ThrottleFlow]
  [EngRunAtv] -> Switch1/2
  Constant3/1 -> Switch1/3
  Switch1/1 -> Core Engine1/1(Engine Speed (RPM))
  [ThrPstCmd_pct] -> Throttle Body1/1(Throttle Position % CMD)
  Core Engine1/3(PE Status) -> Switch16/1
  Core Engine1/4(HC (g/s)) -> Switch12/1
  Core Engine1/1(Brake Torque (Nm)) -> Switch11/1
  Switch16/1 -> [EngPe]
  Crank Process/1(EngActTrq) -> EngEfficiency1/1(Torque), Bus Creator/1  "eng_trq_out_Nm"
  EngEfficiency1/1(PowerLoss) -> EngineThermal1/1(PowerLoss)
  [EngRunAtv] -> Switch11/2, Switch13/2, Switch14/2, Switch16/2, Switch15/2, Switch12/2, Switch9/2
  Switch14/1 -> [EmsNOx]
  Core Engine1/6(NOx (g/s)) -> Switch14/1
  EngineThermal1/1(Temp[degC]) -> [EngTemp]
  Switch13/1 -> [EmsCO]
  [EngSpd_RPM] -> EngEfficiency1/2(Speed)
  Switch9/1 -> [AdvFuelFlowEst], EngEfficiency1/3(Fuel Consumption)  "131"
  Switch15/1 -> [EmsCO2]
  Switch11/1 -> [EngBrkTrq]  "123"
  Switch12/1 -> [EmsHC]
  Core Engine1/7(CO2 (g/s)) -> Switch15/1
  Core Engine1/2(Fuel Flow (g/s)) -> Switch9/1
  Core Engine1/5(CO (g/s)) -> Switch13/1
  Engine Off  1/1 -> Switch9/3, Switch11/3, Switch16/3, Switch15/3, Switch14/3, Switch13/3, Switch12/3
  Engine Inertia/1 -> Bus Creator/2  "eng_inertia_out"
  [EngSpd_RPM] -> Crank Process/5(EngSpd_RPM)
  [EngCrankCmd] -> Crank Process/3(EngCrankCmd)
  Available Fuel/1 -> Crank Process/2(AvlblFuel)
  Bus Creator/1 -> eng_shaft_out/1
  [EngRunAtv] -> Crank Process/1(EngRunAtv)
  [EngShutdown] -> Crank Process/6(EngShutdown)
  [EngBrkTrq] -> Crank Process/4(EngBrkTrq)
  [ThrottleFlow] -> Scope/1
  [MAT] -> Scope1/1
  [MAP] -> Scope2/1
  rad/s to RPM/1 -> max_speed/1
  max_speed/1 -> [EngSpd_RPM], Switch1/1
  Engine Speed (rad/s)/1 -> rad/s to RPM/1
  connections:
  Environment1/LConn1 -- Solver Configuration1/RConn1 -- Exhaust System/RConn1 -- Throttle Body1/LConn1 -- Ambient Air Properties and States1/RConn1
  Throttle Body1/RConn1 -- Intake Manifold1/LConn1 -- Core Engine1/LConn1
  Exhaust System/LConn1 -- Core Engine1/RConn1

== system Clutchless_P2_Parallel_ETE/Camaro Plant Model/ICE Simple1/Engine Plant Modified/ECU Actuators ==
  In1 : Inport
  Bus Selector : BusSelector  OutputSignals=ThrPosCmd_%,Eng12vStrtrMtrCmmdOn,EngRunAtv,FuelPumpEnable,EngShutdown,Eng_Temp,fan_cmd,VehSpdAvgDrvn
  Out1 : Outport
  Out2 : Outport  Port=2
  Out3 : Outport  Port=3
  Out4 : Outport  Port=4
  Out5 : Outport  Port=5
  Out6 : Outport  Port=6
  Out7 : Outport  Port=7
  Out8 : Outport  Port=8
  wires:
  Bus Selector/5 -> Out5/1  "<EngShutdown>"
  Bus Selector/4 -> Out4/1  "<FuelPumpEnable>"
  In1/1 -> Bus Selector/1
  Bus Selector/1 -> Out1/1  "<ThrPosCmd_%>"
  Bus Selector/2 -> Out2/1  "<Eng12vStrtrMtrCmmdOn>"
  Bus Selector/3 -> Out3/1  "<EngRunAtv>"
  Bus Selector/6 -> Out6/1  "<Eng_Temp>"
  Bus Selector/7 -> Out7/1  "<fan_cmd>"
  Bus Selector/8 -> Out8/1  "<VehSpdAvgDrvn>"
